simulink model "ADCS_onOrbit"  (R2024b)
settings: Solver=ode4  StartTime=0.0  StopTime=tspan  FixedStep=1  RelTol=1e-5
values from neighbouring files (symbols this model uses):
  A_list = [10*30; 10*30; 10*10; 10*30; 10*30; 10*10] * 1e-04    [acsLoadParameters.m]
  A_m = eye(3)    [acsLoadParameters.m]
  A_w = eye(3)    [acsLoadParameters.m]
  CD = 2.3    [acsLoadParameters.m]
  COP = [xAxis/2   0          0 ... (first row only)    [acsLoadParameters.m]
  dYear = decyear(YYYY,MM,DD)    [acsLoadParameters.m]
  e = 6.91944e-15    [acsLoadParameters.m]
  eta = 0.3    [acsLoadParameters.m]
  inc = 97.4377    [acsLoadParameters.m]
  J_body = [I_x 0 0; 0 I_y 0; 0 0 I_z]    [acsLoadParameters.m]
  J_wheels = [12894 0 0; 0 12774 0; 0 0 18389] * 1e-09    [acsLoadParameters.m]
  JD0 = juliandate(YYYY,MM,DD,HH,MIN,SEC)    [acsLoadParameters.m]
  K_d = 0.008    [acsLoadParameters.m]
  K_p = 0.003    [acsLoadParameters.m]
  K_w = 50e4    (= 500000)    [acsLoadParameters.m]
  m = 4    [acsLoadParameters.m]
  mag_moment = [0.005; 0.005; 0.005]    [acsLoadParameters.m]
  mu = 398600.4418    [acsLoadParameters.m]
  n_list = [1 0 0; 0 1 0; 0 0 1; -1 0 0; 0 -1 0; 0 0 -1]    [acsLoadParameters.m]
  omega = 0    [acsLoadParameters.m]    (also in orbit_plot_sfcn.m = block.InputPort(4).Data(:))
  p = 0.00000451    (= 4.51e-06)    [acsLoadParameters.m]    (also in cubesat_attitude_sfcn.m = ud.cubePos)
  P_0 = 0.0000001 * eye(7)    [acsLoadParameters.m]
  period = sqrt((4* pi^2 * semimajor_axis^3)/(mu))    [acsLoadParameters.m]
  q_ini = [0; 0; 0; 1]    [acsLoadParameters.m]
  raan = 226.816    [acsLoadParameters.m]
  rE = 6378.14    [acsLoadParameters.m]
  semimajor_axis = rE + h_apogee    (= 6913.14)    [acsLoadParameters.m]
  sigma_B_b = 0.05 * [1; 1; 1]    [acsLoadParameters.m]
  sigma_drift = 0.05 * [1; 1; 1] * 0    [acsLoadParameters.m]
  sigma_n = (0.05) * [1; 1; 1] * 0    [acsLoadParameters.m]
  sigma_S_b = 0.05 * [1; 1; 1]    [acsLoadParameters.m]
  tau = 300    [ATT_EKF_DOT.m]    (also in acsLoadParameters.m)
  true_anomaly = 0.0994843    [acsLoadParameters.m]
  w_b_ini = [0; 0.1; 0.1]    [acsLoadParameters.m]
  w_bias_0 = 0.0001 * [1; 1; 1] * 0    [acsLoadParameters.m]
  w_w_ini = [0; 0; 0]    [acsLoadParameters.m]
  wE = [0 0 15.04*(pi/180)*(1/3600)]    [acsLoadParameters.m]
undefined symbols (not defined in the file or in its folder): WMM2020
libraries: simulink_extras x13, matrix_library x9, sharedtransform x7, aerolibgravity2 x1, aerolibutil x1
(part 2 of 3)

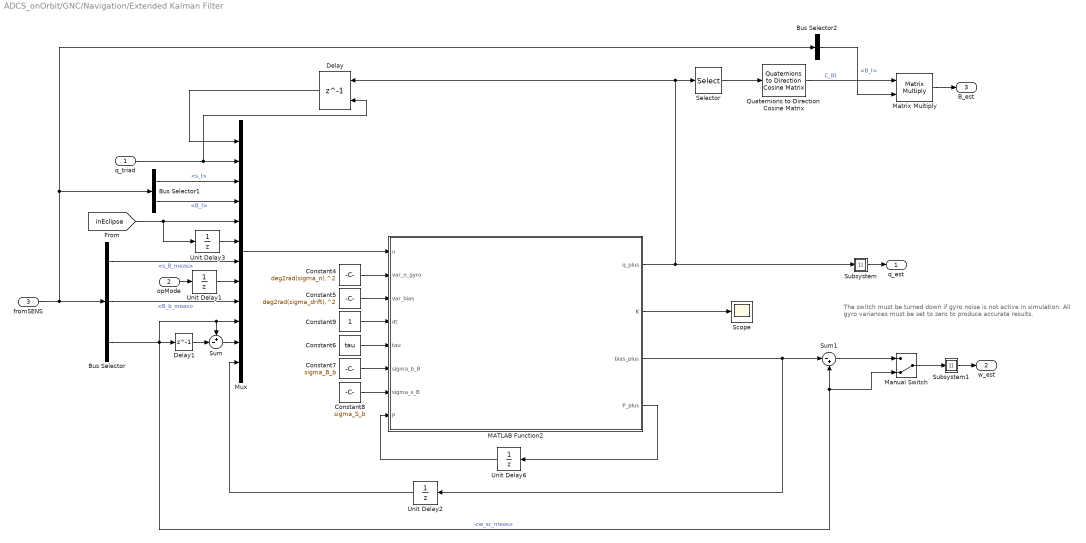
== system ADCS_onOrbit/GNC/Navigation/Extended Kalman Filter ==
  note: The switch must be turned down if gyro noise is not active in simulation.
      | All gyro variances must be set to zero to produce accurate results.
  q_triad : Inport
  opMode : Inport  Port=2
  fromSENS : Inport  Port=3
  Bus Selector : BusSelector  OutputSignals=s_B_meas,B_b_meas,w_sc_meas
  Bus Selector1 : BusSelector  OutputSignals=s_I,B_I
  Bus Selector2 : BusSelector  OutputSignals=B_I
  Constant4 : Constant  Value=deg2rad(sigma_n).^2
  Constant5 : Constant  Value=deg2rad(sigma_drift).^2
  Constant6 : Constant  Value=tau
  Constant7 : Constant  Value=sigma_B_b
  Constant8 : Constant  Value=sigma_S_b
  Constant9 : Constant
  Delay : Delay  DelayLength=1  InitialConditionSource=Input port  InitialCondition=q_ini
      settings: InputPortMap=u0,p4
  Delay1 : Delay  DelayLength=1  InitialCondition=w_b_ini
  MATLAB Function2 : MATLAB Function  TreatAsAtomicUnit=on
  Manual Switch : ManualSwitch  CurrentSetting=0
  Matrix Multiply : Product  Multiplication=Matrix(*)
  Mux : Mux  Inputs=12
  Quaternions to Direction Cosine Matrix : sharedtransform/Quaternions to  Direction Cosine Matrix  aMode=aMode
      settings: LibrarySourceBlock=|
      | aerolibtransform2/Quaternions to
      | Direction Cosine Matrix
  Scope : Scope
  Selector : Selector  InputPortWidth=4  IndexOptions=Index vector (dialog)  Indices=[4 1 2 3]  OutputSizes=1
  Subsystem : Subsystem
  Subsystem1 : Subsystem
  Sum : Sum  Inputs=+-|
  Sum1 : Sum  Inputs=|-+
  Unit Delay1 : UnitDelay  InitialCondition=-1  SampleTime=-1  HasFrameUpgradeWarning=on
  Unit Delay2 : UnitDelay  InitialCondition=w_bias_0  SampleTime=-1  HasFrameUpgradeWarning=on
  Unit Delay3 : UnitDelay  InitialCondition=-1  SampleTime=-1  HasFrameUpgradeWarning=on
  Unit Delay6 : UnitDelay  InitialCondition=P_0  SampleTime=-1  HasFrameUpgradeWarning=on
  q_est : Outport
  w_est : Outport  Port=2
  B_est : Outport  Port=3
  wires:
  [inEclipse] -> Unit Delay3/1, Mux/5
  fromSENS/1 -> Bus Selector1/1, Bus Selector2/1, Bus Selector/1
  MATLAB Function2/1(q_plus) -> Subsystem/1(q), Selector/1, Delay/1
  Sum1/1 -> Manual Switch/1
  Bus Selector/1 -> Mux/7  "<s_B_meas>"
  Bus Selector/2 -> Mux/9  "<B_b_meas>"
  Bus Selector1/1 -> Mux/3  "<s_I>"
  Bus Selector1/2 -> Mux/4  "<B_I>"
  Unit Delay3/1 -> Mux/6
  Delay/1 -> Mux/1
  q_triad/1 -> Delay/2, Mux/2
  opMode/1 -> Unit Delay1/1
  Unit Delay1/1 -> Mux/8
  Bus Selector/3 -> Delay1/1, Sum1/2, Manual Switch/2, Sum/1, Mux/10  "<w_sc_meas>"
  Sum/1 -> Mux/11
  Delay1/1 -> Sum/2
  MATLAB Function2/3(bias_plus) -> Unit Delay2/1, Sum1/1
  Unit Delay2/1 -> Mux/12
  Mux/1 -> MATLAB Function2/1(u)
  MATLAB Function2/4(P_plus) -> Unit Delay6/1
  Constant4/1 -> MATLAB Function2/2(var_n_gyro)
  Constant5/1 -> MATLAB Function2/3(var_bias)
  Constant6/1 -> MATLAB Function2/5(tau)
  Constant7/1 -> MATLAB Function2/6(sigma_b_B)
  Constant8/1 -> MATLAB Function2/7(sigma_s_B)
  Constant9/1 -> MATLAB Function2/4(dt)
  MATLAB Function2/2(K) -> Scope/1
  Selector/1 -> Quaternions to Direction Cosine Matrix/1
  Quaternions to Direction Cosine Matrix/1 -> Matrix Multiply/1  "C_BI"
  Bus Selector2/1 -> Matrix Multiply/2  "<B_I>"
  Matrix Multiply/1 -> B_est/1
  Subsystem/1(Out1) -> q_est/1
  Subsystem1/1(Out1) -> w_est/1
  Unit Delay6/1 -> MATLAB Function2/8(P)
  Manual Switch/1 -> Subsystem1/1(In1)

== system ADCS_onOrbit/GNC/Navigation/TRIAD Determination ==
  fromSENS : Inport
  Bus Selector : BusSelector  OutputSignals=s_I,B_I,s_B_meas,B_b_meas
  Direction Cosine Matrix to Quaternions : sharedtransform/Direction Cosine Matrix  to Quaternions  aMode=0  action=None  tolerance=eps(2)
      settings: LibrarySourceBlock=|
      | aerolibtransform2/Direction Cosine Matrix
      | to Quaternions
  MATLAB Function1 : MATLAB Function  TreatAsAtomicUnit=on
  Quaternion Continuity : Subsystem
      mask Display: disp('Quaternion\nContinuity');
  Selector2 : Selector  InputPortWidth=4  IndexOptions=Index vector (dialog)  Indices=[2 3 4 1]  OutputSizes=1
  q_det : Outport
  wires:
  Bus Selector/3 -> MATLAB Function1/3(s_b)  "<s_B_meas>"
  Bus Selector/4 -> MATLAB Function1/4(m_b)  "<B_b_meas>"
  fromSENS/1 -> Bus Selector/1
  MATLAB Function1/1(C_BI) -> Direction Cosine Matrix to Quaternions/1
  Direction Cosine Matrix to Quaternions/1 -> Selector2/1
  Selector2/1 -> Quaternion Continuity/1(q)
  Quaternion Continuity/1(q_smooth) -> q_det/1
  Bus Selector/1 -> MATLAB Function1/1(s_I)  "<s_I>"
  Bus Selector/2 -> MATLAB Function1/2(m_I)  "<B_I>"

== system ADCS_onOrbit/GNC/Navigation/rad2deg ==
  In1 : Inport
  Gain : Gain  Gain=57.2958
  Out1 : Outport
  wires:
  In1/1 -> Gain/1
  Gain/1 -> Out1/1

== system ADCS_onOrbit/RWP/Environment/Variant Subsystem ==
  note: 1) Add Subsystem or Model blocks as valid variant choices.
      | 2) You cannot connect blocks at this level. At simulation, connectivity is automatically
      | determined, based on the active variant and port name matching.
  C_BI : Inport
  s : Inport  Port=2
  state : Inport  Port=3
  ENV : Subsystem  VariantControl=external_torques == true
  noENV : Subsystem  VariantControl=external_torques == false
  B_b : Outport
  T_ext : Outport  Port=2
  a_drag : Outport  Port=3
  B_I : Outport  Port=4

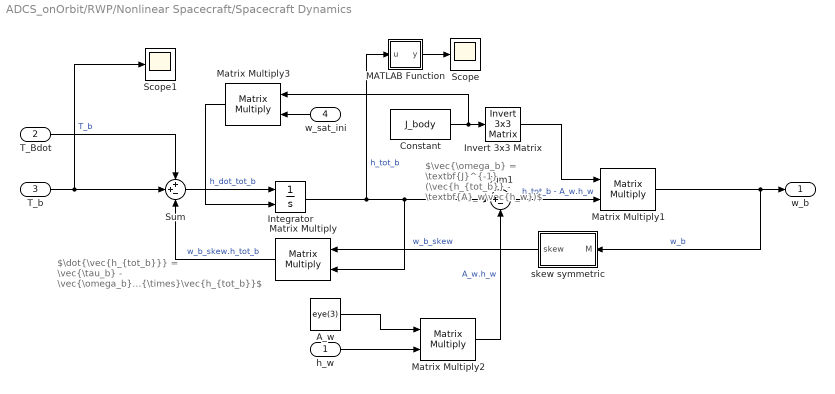
== system ADCS_onOrbit/RWP/Nonlinear Spacecraft/Spacecraft Dynamics ==
  note: $\dot{\vec{h_{tot_b}}} = \vec{\tau_b} - \vec{\omega_b}^{\times}\vec{h_{tot_b}}$
  note: $\vec{\omega_b} = \textbf{J}^{-1} (\vec{h_{tot_b}} - \textbf{A}_w\vec{h_w})$
  h_w : Inport
  T_Bdot : Inport  Port=2
  T_b : Inport  Port=3
  w_sat_ini : Inport  Port=4
  A_w : Constant  Value=eye(3)  VectorParams1D=off
  Constant : Constant  Value=J_body
  Integrator : Integrator  InitialConditionSource=external
  Invert 3x3 Matrix : aerolibutil/Invert  3x3 Matrix
  MATLAB Function : MATLAB Function  TreatAsAtomicUnit=on
  Matrix Multiply{,1..3} (4 alike) : Product  Multiplication=Matrix(*)
  Scope : Scope
  Scope1 : Scope
  Sum : Sum  Inputs=++-
  Sum1 : Sum  Inputs=|+-
  skew symmetric : MATLAB Function  TreatAsAtomicUnit=on
  w_b : Outport
  wires:
  Matrix Multiply2/1 -> Sum1/2  "A_w.h_w"
  A_w/1 -> Matrix Multiply2/1
  skew symmetric/1(skew) -> Matrix Multiply/1  "w_b_skew"
  Matrix Multiply1/1 -> w_b/1, skew symmetric/1(M)  "w_b"
  Invert 3x3 Matrix/1 -> Matrix Multiply1/1
  Constant/1 -> Matrix Multiply3/1, Invert 3x3 Matrix/1
  Sum1/1 -> Matrix Multiply1/2  "h_tot_b - A_w.h_w"
  h_w/1 -> Matrix Multiply2/2
  T_b/1 -> Scope1/1, Sum/2  "T_b"
  Matrix Multiply/1 -> Sum/3  "w_b_skew.h_tot_b"
  Sum/1 -> Integrator/1  "h_dot_tot_b"
  Integrator/1 -> MATLAB Function/1(u), Sum1/1, Matrix Multiply/2  "h_tot_b"
  w_sat_ini/1 -> Matrix Multiply3/2
  Matrix Multiply3/1 -> Integrator/2
  T_Bdot/1 -> Sum/1
  MATLAB Function/1(y) -> Scope/1

== system ADCS_onOrbit/RWP/Nonlinear Spacecraft/Spacecraft Kinematics ==
  note: Quaternion Kinematics Equation:
      | $\dot{\textbf{q}} = \frac{1}{2} \Omega (\vec\omega) \textbf{q}$
  w : Inport
  q_ini : Inport  Port=2
  Gain : Gain  Gain=1/2
  Integrator1 : Integrator  InitialConditionSource=external  InitialCondition=[1 0 0 0]
  MATLAB Function : MATLAB Function  TreatAsAtomicUnit=on
  Matrix Multiply3 : Product  Multiplication=Matrix(*)
  Quaternion Normalize : MATLAB Function  TreatAsAtomicUnit=on
  q : Outport
  wires:
  Matrix Multiply3/1 -> Integrator1/1  "dq/dt"
  MATLAB Function/1(OMEGA) -> Matrix Multiply3/1
  Gain/1 -> Matrix Multiply3/2
  q_ini/1 -> Integrator1/2
  Integrator1/1 -> Quaternion Normalize/1(q)  "q"
  w/1 -> MATLAB Function/1(w)
  Quaternion Normalize/1(q_norm) -> q/1, Gain/1

== system ADCS_onOrbit/RWP/Nonlinear Spacecraft/Subsystem ==
  q : Inport
  MATLAB Function : MATLAB Function  TreatAsAtomicUnit=on
  Radians to Degrees : simulink_extras/Transformations/Radians to Degrees
  Radians to Degrees1 : simulink_extras/Transformations/Radians to Degrees
  Radians to Degrees2 : simulink_extras/Transformations/Radians to Degrees
  To Workspace : ToWorkspace  VariableName=roll  SampleTime=-1
  To Workspace1 : ToWorkspace  VariableName=pitch  SampleTime=-1
  To Workspace2 : ToWorkspace  VariableName=yaw  SampleTime=-1
  Out1 : Outport
  tag scope: scAtt=global
  wires:
  q/1 -> MATLAB Function/1(q), Out1/1, [scAtt]
  MATLAB Function/3(pitch) -> Radians to Degrees1/1
  Radians to Degrees2/1 -> To Workspace2/1
  MATLAB Function/4(yaw) -> Radians to Degrees2/1
  MATLAB Function/2(roll) -> Radians to Degrees/1
  Radians to Degrees/1 -> To Workspace/1
  Radians to Degrees1/1 -> To Workspace1/1

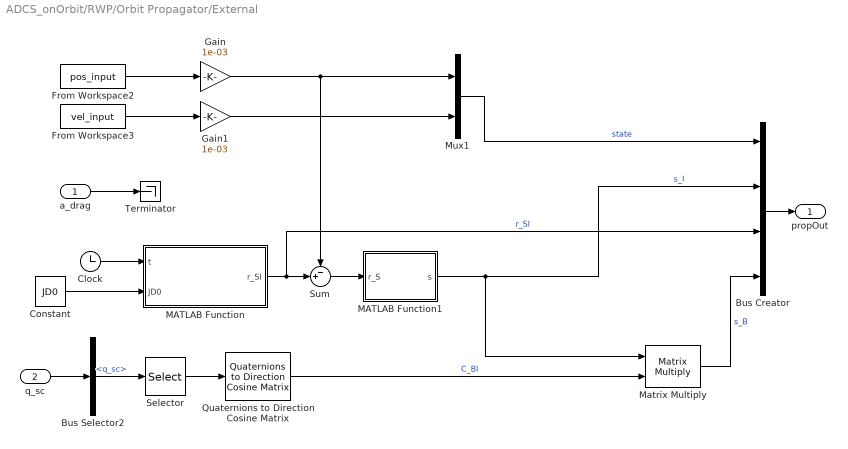
== system ADCS_onOrbit/RWP/Orbit Propagator/External ==
  a_drag : Inport
  q_sc : Inport  Port=2
  Bus Creator : BusCreator  Inputs=4
  Bus Selector2 : BusSelector  OutputSignals=q_sc
  Clock : Clock
  Constant : Constant  Value=JD0
  From Workspace2 : FromWorkspace  VariableName=pos_input
  From Workspace3 : FromWorkspace  VariableName=vel_input
  Gain : Gain  Gain=1e-03
  Gain1 : Gain  Gain=1e-03
  MATLAB Function : MATLAB Function  TreatAsAtomicUnit=on
  MATLAB Function1 : MATLAB Function  TreatAsAtomicUnit=on
  Matrix Multiply : Product  Multiplication=Matrix(*)
  Mux1 : Mux  Inputs=2
  Quaternions to Direction Cosine Matrix : sharedtransform/Quaternions to  Direction Cosine Matrix  aMode=aMode
      settings: LibrarySourceBlock=|
      | aerolibtransform2/Quaternions to
      | Direction Cosine Matrix
  Selector : Selector  InputPortWidth=4  IndexOptions=Index vector (dialog)  Indices=[4 1 2 3]  OutputSizes=1
  Sum : Sum  Inputs=-+|
  Terminator : Terminator
  propOut : Outport
  wires:
  Clock/1 -> MATLAB Function/1(t)
  From Workspace3/1 -> Gain1/1
  Gain/1 -> Sum/1, Mux1/1
  From Workspace2/1 -> Gain/1
  Sum/1 -> MATLAB Function1/1(r_S)
  Constant/1 -> MATLAB Function/2(JD0)
  Gain1/1 -> Mux1/2
  a_drag/1 -> Terminator/1
  MATLAB Function/1(r_SI) -> Bus Creator/3, Sum/2  "r_SI"
  MATLAB Function1/1(s) -> Matrix Multiply/1, Bus Creator/2  "s_I"
  Matrix Multiply/1 -> Bus Creator/4  "s_B"
  Bus Creator/1 -> propOut/1
  Mux1/1 -> Bus Creator/1  "state"
  Quaternions to Direction Cosine Matrix/1 -> Matrix Multiply/2  "C_BI"
  Selector/1 -> Quaternions to Direction Cosine Matrix/1
  q_sc/1 -> Bus Selector2/1
  Bus Selector2/1 -> Selector/1  "<q_sc>"

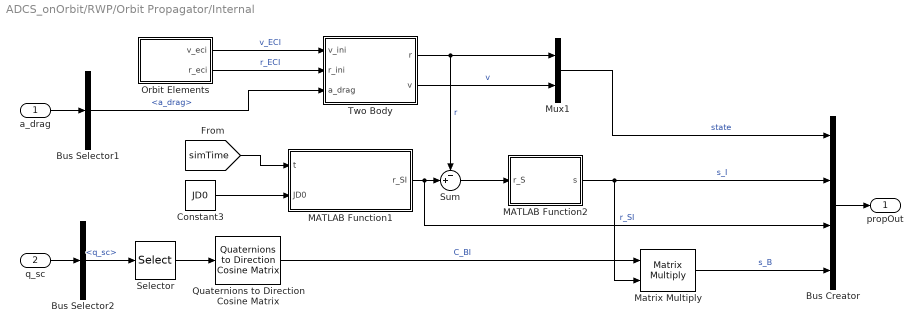
== system ADCS_onOrbit/RWP/Orbit Propagator/Internal ==
  a_drag : Inport
  q_sc : Inport  Port=2
  Bus Creator : BusCreator  Inputs=4
  Bus Selector1 : BusSelector  OutputSignals=a_drag
  Bus Selector2 : BusSelector  OutputSignals=q_sc
  Constant3 : Constant  Value=JD0
  MATLAB Function1 : MATLAB Function  TreatAsAtomicUnit=on
  MATLAB Function2 : MATLAB Function  TreatAsAtomicUnit=on
  Matrix Multiply : Product  Multiplication=Matrix(*)
  Mux1 : Mux  Inputs=2
  Orbit Elements : Subsystem
      mask Display: disp('OE2rv');
  Quaternions to Direction Cosine Matrix : sharedtransform/Quaternions to  Direction Cosine Matrix  aMode=aMode
      settings: LibrarySourceBlock=|
      | aerolibtransform2/Quaternions to
      | Direction Cosine Matrix
  Selector : Selector  InputPortWidth=4  IndexOptions=Index vector (dialog)  Indices=[4 1 2 3]  OutputSizes=1
  Sum : Sum  Inputs=-+|
  Two Body : Subsystem
      mask Display: disp('Two Body');
  propOut : Outport
  wires:
  Mux1/1 -> Bus Creator/1  "state"
  MATLAB Function1/1(r_SI) -> Bus Creator/3, Sum/2  "r_SI"
  Constant3/1 -> MATLAB Function1/2(JD0)
  [simTime] -> MATLAB Function1/1(t)
  Sum/1 -> MATLAB Function2/1(r_S)
  Orbit Elements/2(r_eci) -> Two Body/2(r_ini)  "r_ECI"
  Two Body/2(v) -> Mux1/2  "v"
  Two Body/1(r) -> Mux1/1, Sum/1  "r"
  a_drag/1 -> Bus Selector1/1
  Orbit Elements/1(v_eci) -> Two Body/1(v_ini)  "v_ECI"
  q_sc/1 -> Bus Selector2/1
  Selector/1 -> Quaternions to Direction Cosine Matrix/1
  Quaternions to Direction Cosine Matrix/1 -> Matrix Multiply/1  "C_BI"
  MATLAB Function2/1(s) -> Matrix Multiply/2, Bus Creator/2  "s_I"
  Matrix Multiply/1 -> Bus Creator/4  "s_B"
  Bus Selector2/1 -> Selector/1  "<q_sc>"
  Bus Selector1/1 -> Two Body/3(a_drag)  "<a_drag>"
  Bus Creator/1 -> propOut/1

== system ADCS_onOrbit/RWP/Subsystem/Subsystem1 ==
  In1 : Inport
  Out1 : Outport
  tag scope: w_w=global
  wires:
  In1/1 -> Out1/1, [w_w]

== system ADCS_onOrbit/RWP/Subsystem/Subsystem2 ==
  In1 : Inport
  Out1 : Outport
  tag scope: s_I=global
  wires:
  In1/1 -> [s_I], Out1/1

== system ADCS_onOrbit/GNC/Guidance/Nadir Pointing/Quaternion Continuity ==
  q : Inport
  MATLAB Function2 : MATLAB Function  TreatAsAtomicUnit=on
  Unit Delay1 : UnitDelay  InitialCondition=[0 0 0 1]'  SampleTime=-1  HasFrameUpgradeWarning=on
  q_smooth : Outport
  wires:
  MATLAB Function2/1(q_smooth) -> q_smooth/1, Unit Delay1/1
  Unit Delay1/1 -> MATLAB Function2/2(q_prev)
  q/1 -> MATLAB Function2/1(q)

== system ADCS_onOrbit/GNC/Guidance/Sun Pointing/Quaternion Continuity ==
  q : Inport
  MATLAB Function2 : MATLAB Function  TreatAsAtomicUnit=on
  Unit Delay1 : UnitDelay  InitialCondition=[0 0 0 1]'  SampleTime=-1  HasFrameUpgradeWarning=on
  q_smooth : Outport
  wires:
  MATLAB Function2/1(q_smooth) -> q_smooth/1, Unit Delay1/1
  Unit Delay1/1 -> MATLAB Function2/2(q_prev)
  q/1 -> MATLAB Function2/1(q)

== system ADCS_onOrbit/GNC/Guidance/Target Pointing/Quaternion Continuity ==
  q : Inport
  MATLAB Function2 : MATLAB Function  TreatAsAtomicUnit=on
  Unit Delay1 : UnitDelay  InitialCondition=[0 0 0 1]'  SampleTime=-1  HasFrameUpgradeWarning=on
  q_smooth : Outport
  wires:
  MATLAB Function2/1(q_smooth) -> q_smooth/1, Unit Delay1/1
  Unit Delay1/1 -> MATLAB Function2/2(q_prev)
  q/1 -> MATLAB Function2/1(q)

== system ADCS_onOrbit/GNC/Navigation/Extended Kalman Filter/Subsystem ==
  q : Inport
  MATLAB Function : MATLAB Function  TreatAsAtomicUnit=on
  Radians to Degrees : simulink_extras/Transformations/Radians to Degrees
  Radians to Degrees1 : simulink_extras/Transformations/Radians to Degrees
  Radians to Degrees2 : simulink_extras/Transformations/Radians to Degrees
  To Workspace : ToWorkspace  VariableName=rollEKF  SampleTime=-1
  To Workspace1 : ToWorkspace  VariableName=pitchEKF  SampleTime=-1
  To Workspace2 : ToWorkspace  VariableName=yawEKF  SampleTime=-1
  Out1 : Outport
  tag scope: rpy=global
  wires:
  q/1 -> MATLAB Function/1(q), Out1/1
  MATLAB Function/3(pitch) -> Radians to Degrees1/1
  Radians to Degrees2/1 -> To Workspace2/1
  MATLAB Function/4(yaw) -> Radians to Degrees2/1
  MATLAB Function/2(roll) -> Radians to Degrees/1
  Radians to Degrees/1 -> To Workspace/1
  Radians to Degrees1/1 -> To Workspace1/1
  MATLAB Function/1(rpy) -> [rpy]  "rpy"

== system ADCS_onOrbit/GNC/Navigation/Extended Kalman Filter/Subsystem1 ==
  In1 : Inport
  Out1 : Outport
  tag scope: w_body=global
  wires:
  In1/1 -> Out1/1, [w_body]

== system ADCS_onOrbit/GNC/Navigation/TRIAD Determination/Quaternion Continuity ==
  q : Inport
  MATLAB Function2 : MATLAB Function  TreatAsAtomicUnit=on
  Unit Delay1 : UnitDelay  InitialCondition=[0 0 0 1]'  SampleTime=-1  HasFrameUpgradeWarning=on
  q_smooth : Outport
  wires:
  MATLAB Function2/1(q_smooth) -> q_smooth/1, Unit Delay1/1
  Unit Delay1/1 -> MATLAB Function2/2(q_prev)
  q/1 -> MATLAB Function2/1(q)

== system ADCS_onOrbit/RWP/Environment/Variant Subsystem/ENV ==
  C_BI : Inport
  s : Inport  Port=2
  state : Inport  Port=3
  Drag : Subsystem
  Gravity Gradient : Subsystem
  Mag Torque : Subsystem
  Selector : Selector  InputPortWidth=6  IndexOptions=Index vector (dialog)  Indices=[1 2 3]  OutputSizes=1
  Selector1 : Selector  InputPortWidth=6  IndexOptions=Index vector (dialog)  Indices=[4 5 6]  OutputSizes=1
  Solar Radiation Pressure : Subsystem
  Sum : Sum  Inputs=++++
  B_b : Outport
  T_ext : Outport  Port=2
  a_drag : Outport  Port=3
  B_I : Outport  Port=4
  wires:
  Drag/2(a_drag) -> a_drag/1
  C_BI/1 -> Solar Radiation Pressure/1(C_BI), Drag/3(C_BI), Gravity Gradient/2(C_BI), Mag Torque/2(C_BI)
  Selector1/1 -> Drag/2(v_ECI)  "vel"
  Gravity Gradient/1(T_g) -> Sum/3
  Sum/1 -> T_ext/1  "External Torque"
  Mag Torque/1(T_mag) -> Sum/4
  Drag/1(T_atm) -> Sum/2
  Selector/1 -> Drag/1(r_ECI), Gravity Gradient/1(r_ECI), Mag Torque/1(r_ECI)  "pos"
  s/1 -> Solar Radiation Pressure/2(s)
  Mag Torque/2(B_b) -> B_b/1
  Solar Radiation Pressure/1(T_SRP) -> Sum/1
  state/1 -> Selector1/1, Selector/1
  Mag Torque/3(B_I) -> B_I/1

== system ADCS_onOrbit/RWP/Environment/Variant Subsystem/noENV ==
  C_BI : Inport
  s : Inport  Port=2
  state : Inport  Port=3
  Constant : Constant  Value=[0; 0; 0]  VectorParams1D=off
  Constant1 : Constant  Value=[0; 0; 0]
  Mag Torque : Subsystem
  Selector : Selector  InputPortWidth=6  IndexOptions=Index vector (dialog)  Indices=[1 2 3]  OutputSizes=1
  Terminator : Terminator
  Terminator1 : Terminator
  B_b : Outport
  T_ext : Outport  Port=2
  a_drag : Outport  Port=3
  B_I : Outport  Port=4
  wires:
  Constant1/1 -> a_drag/1
  Mag Torque/1(T_mag) -> Terminator1/1
  s/1 -> Terminator/1
  C_BI/1 -> Mag Torque/2(C_BI)
  Selector/1 -> Mag Torque/1(r_ECI)  "pos"
  state/1 -> Selector/1
  Constant/1 -> T_ext/1
  Mag Torque/2(B_b) -> B_b/1
  Mag Torque/3(B_I) -> B_I/1

== system ADCS_onOrbit/RWP/Orbit Propagator/Internal/Orbit Elements ==
  Constant : Constant  Value=semimajor_axis
  Constant1 : Constant  Value=e
  Constant2 : Constant  Value=inc
  Constant3 : Constant  Value=raan
  Constant4 : Constant  Value=omega
  Constant5 : Constant  Value=true_anomaly
  Constant6 : Constant  Value=mu
  Degrees to Radians{,1..3} (4 alike) : simulink_extras/Transformations/Degrees to Radians
  oe2rv : MATLAB Function  TreatAsAtomicUnit=on
  v_eci : Outport
  r_eci : Outport  Port=2
  wires:
  Degrees to Radians1/1 -> oe2rv/4(RAAN)
  Constant3/1 -> Degrees to Radians1/1
  Constant1/1 -> oe2rv/2(e)
  Degrees to Radians3/1 -> oe2rv/6(nu)
  Constant5/1 -> Degrees to Radians3/1
  Constant2/1 -> Degrees to Radians/1
  Constant4/1 -> Degrees to Radians2/1
  Degrees to Radians/1 -> oe2rv/3(i)
  Degrees to Radians2/1 -> oe2rv/5(omega)
  oe2rv/1(r_eci) -> r_eci/1
  oe2rv/2(v_eci) -> v_eci/1
  Constant/1 -> oe2rv/1(a)
  Constant6/1 -> oe2rv/7(mu)

== system ADCS_onOrbit/RWP/Orbit Propagator/Internal/Two Body ==
  v_ini : Inport
  r_ini : Inport  Port=2
  a_drag : Inport  Port=3
  Constant : Constant  Value=mu
  Constant1 : Constant  Value=rE
  Integrator2 : Integrator  InitialConditionSource=external
  Integrator3 : Integrator  InitialConditionSource=external
  MATLAB Function1 : MATLAB Function  TreatAsAtomicUnit=on
  MATLAB Function3 : MATLAB Function  TreatAsAtomicUnit=on
  Sum1 : Sum  Inputs=+++
  r : Outport
  v : Outport  Port=2
  wires:
  Constant/1 -> MATLAB Function3/2(mu), MATLAB Function1/2(mu)
  v_ini/1 -> Integrator2/2
  Integrator2/1 -> Integrator3/1, v/1  "r"
  r_ini/1 -> Integrator3/2
  MATLAB Function3/1(a_j2) -> Sum1/3  "a_J2"
  MATLAB Function1/1(a_I) -> Sum1/2
  Sum1/1 -> Integrator2/1
  Integrator3/1 -> r/1, MATLAB Function1/1(r_I), MATLAB Function3/1(r)  "r"
  a_drag/1 -> Sum1/1
  Constant1/1 -> MATLAB Function3/3(rE)

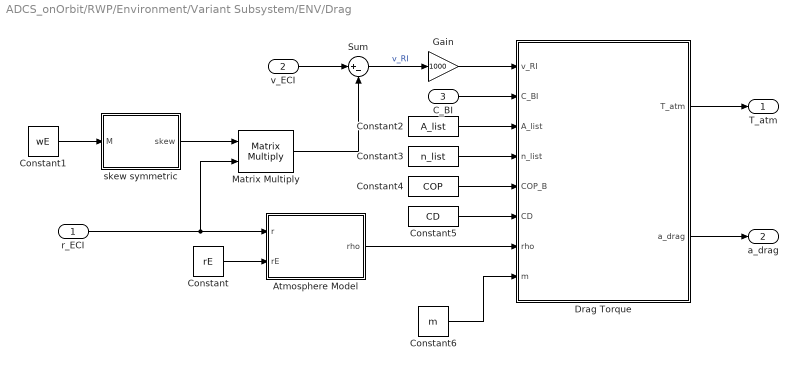
== system ADCS_onOrbit/RWP/Environment/Variant Subsystem/ENV/Drag ==
  r_ECI : Inport
  v_ECI : Inport  Port=2
  C_BI : Inport  Port=3
  Atmosphere Model : MATLAB Function  TreatAsAtomicUnit=on
  Constant : Constant  Value=rE
  Constant1 : Constant  Value=wE
  Constant2 : Constant  Value=A_list
  Constant3 : Constant  Value=n_list
  Constant4 : Constant  Value=COP
  Constant5 : Constant  Value=CD
  Constant6 : Constant  Value=m
  Drag Torque : MATLAB Function  TreatAsAtomicUnit=on
  Gain : Gain  Gain=1000
  Matrix Multiply : Product  Multiplication=Matrix(*)
  Sum : Sum  Inputs=|+-
  skew symmetric : MATLAB Function  TreatAsAtomicUnit=on
  T_atm : Outport
  a_drag : Outport  Port=2
  wires:
  Drag Torque/2(a_drag) -> a_drag/1
  Constant6/1 -> Drag Torque/8(m)
  Atmosphere Model/1(rho) -> Drag Torque/7(rho)
  Constant5/1 -> Drag Torque/6(CD)
  Constant4/1 -> Drag Torque/5(COP_B)
  Constant3/1 -> Drag Torque/4(n_list)
  Constant2/1 -> Drag Torque/3(A_list)
  C_BI/1 -> Drag Torque/2(C_BI)
  Gain/1 -> Drag Torque/1(v_RI)
  Sum/1 -> Gain/1  "v_RI"
  v_ECI/1 -> Sum/1
  Matrix Multiply/1 -> Sum/2
  Drag Torque/1(T_atm) -> T_atm/1
  skew symmetric/1(skew) -> Matrix Multiply/1
  Constant1/1 -> skew symmetric/1(M)
  Constant/1 -> Atmosphere Model/2(rE)
  r_ECI/1 -> Atmosphere Model/1(r), Matrix Multiply/2

== system ADCS_onOrbit/RWP/Environment/Variant Subsystem/ENV/Gravity Gradient ==
  r_ECI : Inport
  C_BI : Inport  Port=2
  Constant : Constant  Value=J_body
  Constant1 : Constant  Value=mu
  MATLAB Function : MATLAB Function  TreatAsAtomicUnit=on
  Matrix Multiply : Product  Multiplication=Matrix(*)
  Matrix Multiply1 : Product  Multiplication=Matrix(*)
  Matrix Multiply2 : Product  Multiplication=Matrix(*)
  Reshape1 : Reshape  OutputDimensionality=Customize  OutputDimensions=[3,1]
  skew symmetric : MATLAB Function  TreatAsAtomicUnit=on
  T_g : Outport
  wires:
  MATLAB Function/1(T_g) -> T_g/1
  Constant1/1 -> MATLAB Function/2(mu)
  Matrix Multiply2/1 -> MATLAB Function/3(r_skew_J_r)
  Matrix Multiply1/1 -> Matrix Multiply2/1
  Constant/1 -> Matrix Multiply1/2
  skew symmetric/1(skew) -> Matrix Multiply1/1
  C_BI/1 -> Matrix Multiply/1
  r_ECI/1 -> Matrix Multiply/2
  Matrix Multiply/1 -> Reshape1/1
  Reshape1/1 -> skew symmetric/1(M), MATLAB Function/1(r), Matrix Multiply2/2

== system ADCS_onOrbit/RWP/Environment/Variant Subsystem/ENV/Mag Torque ==
  r_ECI : Inport
  C_BI : Inport  Port=2
  Constant : Constant  Value=wE
  Constant1 : Constant  Value=dYear
  Constant4 : Constant  Value=mag_moment
  Demux1 : Demux  Outputs=2
  ECEF Position to LLA : ECEF2LLA
  Gain3 : Gain  Gain=1000
  MATLAB Function : MATLAB Function  TreatAsAtomicUnit=on
  MATLAB Function1 : MATLAB Function  TreatAsAtomicUnit=on
  Matrix Multiply : Product  Multiplication=Matrix(*)
  Subsystem2 : Subsystem
  T_mag : Outport
  B_b : Outport  Port=2
  B_I : Outport  Port=3
  wires:
  C_BI/1 -> MATLAB Function1/6(C_BI)
  Gain3/1 -> ECEF Position to LLA/1
  Matrix Multiply/1 -> Gain3/1
  r_ECI/1 -> Matrix Multiply/2
  MATLAB Function/1(C_IF) -> Matrix Multiply/1, Subsystem2/1(In1)
  Constant/1 -> MATLAB Function/1(wE)
  [simTime] -> MATLAB Function/2(t)
  ECEF Position to LLA/1 -> Demux1/1
  Demux1/1 -> MATLAB Function1/1(lat)
  Demux1/2 -> MATLAB Function1/2(lon)
  ECEF Position to LLA/2 -> MATLAB Function1/3(h)
  Constant1/1 -> MATLAB Function1/4(dYear)
  Constant4/1 -> MATLAB Function1/7(m)
  MATLAB Function1/1(b_I) -> B_I/1
  MATLAB Function1/2(b_B) -> B_b/1
  MATLAB Function1/3(T_m) -> T_mag/1
  Subsystem2/1(Out1) -> MATLAB Function1/5(C_IF)

== system ADCS_onOrbit/RWP/Environment/Variant Subsystem/ENV/Solar Radiation Pressure ==
  C_BI : Inport
  s : Inport  Port=2
  Constant1 : Constant  Value=p
  Constant2 : Constant  Value=eta
  Constant3 : Constant  Value=A_list
  Constant4 : Constant  Value=n_list
  Constant5 : Constant  Value=COP
  MATLAB Function2 : MATLAB Function  TreatAsAtomicUnit=on
  T_SRP : Outport
  wires:
  MATLAB Function2/1(T_SRP) -> T_SRP/1
  C_BI/1 -> MATLAB Function2/7(C_BI)
  Constant5/1 -> MATLAB Function2/6(COP)
  Constant4/1 -> MATLAB Function2/5(n_list)
  Constant3/1 -> MATLAB Function2/4(A_list)
  Constant2/1 -> MATLAB Function2/3(eta)
  Constant1/1 -> MATLAB Function2/2(p)
  s/1 -> MATLAB Function2/1(r_sun)

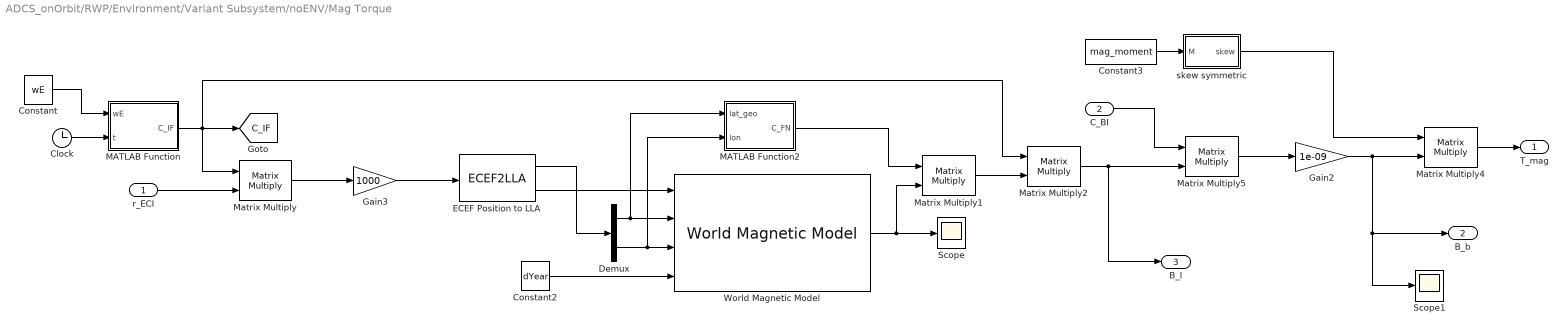
== system ADCS_onOrbit/RWP/Environment/Variant Subsystem/noENV/Mag Torque ==
  r_ECI : Inport
  C_BI : Inport  Port=2
  Clock : Clock
  Constant : Constant  Value=wE
  Constant2 : Constant  Value=dYear
  Constant3 : Constant  Value=mag_moment
  Demux : Demux  Outputs=2
  ECEF Position to LLA : ECEF2LLA
  Gain2 : Gain  Gain=1e-09
  Gain3 : Gain  Gain=1000
  MATLAB Function : MATLAB Function  TreatAsAtomicUnit=on
  MATLAB Function2 : MATLAB Function  TreatAsAtomicUnit=on
  Matrix Multiply{,1..2,4..5} (5 alike) : Product  Multiplication=Matrix(*)
  Scope : Scope
  Scope1 : Scope
  World Magnetic Model : aerolibgravity2/World Magnetic Model  model=WMM2020 (2020-2025)  customFile='WMM2020.COF'  units=Metric (MKS)  time_in=on  month=January  day=1  year=2020  action=Error  h_out=off  dec_out=off  inc_out=off  ti_out=off
  skew symmetric : MATLAB Function  TreatAsAtomicUnit=on
  T_mag : Outport
  B_b : Outport  Port=2
  B_I : Outport  Port=3
  tag scope: C_IF=global
  wires:
  Matrix Multiply5/1 -> Gain2/1
  C_BI/1 -> Matrix Multiply5/1
  Gain3/1 -> ECEF Position to LLA/1
  Demux/2 -> World Magnetic Model/3, MATLAB Function2/2(lon)
  Demux/1 -> World Magnetic Model/2, MATLAB Function2/1(lat_geo)
  ECEF Position to LLA/2 -> World Magnetic Model/1
  ECEF Position to LLA/1 -> Demux/1
  Matrix Multiply4/1 -> T_mag/1
  skew symmetric/1(skew) -> Matrix Multiply4/1
  Gain2/1 -> Matrix Multiply4/2, Scope1/1, B_b/1
  Constant3/1 -> skew symmetric/1(M)
  Matrix Multiply2/1 -> B_I/1, Matrix Multiply5/2
  Matrix Multiply1/1 -> Matrix Multiply2/2
  MATLAB Function2/1(C_FN) -> Matrix Multiply1/1
  World Magnetic Model/1 -> Scope/1, Matrix Multiply1/2
  Constant2/1 -> World Magnetic Model/4
  Matrix Multiply/1 -> Gain3/1
  r_ECI/1 -> Matrix Multiply/2
  MATLAB Function/1(C_IF) -> [C_IF], Matrix Multiply/1, Matrix Multiply2/1
  Constant/1 -> MATLAB Function/1(wE)
  Clock/1 -> MATLAB Function/2(t)

== system ADCS_onOrbit/RWP/Environment/Variant Subsystem/ENV/Mag Torque/Subsystem2 ==
  In1 : Inport
  Out1 : Outport
  tag scope: C_IF=global
  wires:
  In1/1 -> [C_IF], Out1/1

== matlab function ADCS_onOrbit/GNC/Guidance/Nadir Pointing/Quaternion Continuity/MATLAB Function2 ==
  data: q input; q_smooth output; q_prev input
function q_smooth = continuity(q, q_prev)

    if dot(q, q_prev) < 0
        q_smooth = -q;
    else
        q_smooth = q;
    end
end

== matlab function ADCS_onOrbit/GNC/Guidance/Sun Pointing/Quaternion Continuity/MATLAB Function2 ==
  data: q input; q_smooth output; q_prev input
function q_smooth = continuity(q, q_prev)

    if dot(q, q_prev) < 0
        q_smooth = -q;
    else
        q_smooth = q;
    end
end

== matlab function ADCS_onOrbit/RWP/Nonlinear Spacecraft/Spacecraft Kinematics/MATLAB Function ==
  data: w input; OMEGA output
function OMEGA = skew(w)

    w_1 = w(1,:);
    w_2 = w(2,:);
    w_3 = w(3,:);

    OMEGA = [0 w_3 -w_2 w_1
            -w_3 0 w_1 w_2
            w_2 -w_1 0 w_3
            -w_1 -w_2 -w_3 0];

end

== matlab function ADCS_onOrbit/GNC/Guidance/Target Pointing/MATLAB Function2 ==
  data: los input; C_BI output; r input; v input
function C_BI = fcn(los, r, v)

    los = los / norm(los);
    
    z_orb = los;

    y_orb = cross(v, r) / norm(cross(v,r)); % orbit normal
    y_orb = y_orb / norm(y_orb);

    x_orb = cross(y_orb, z_orb); 
    x_orb = x_orb / norm(x_orb);
    
    C_BI = [x_orb, y_orb, z_orb]';

end

== matlab function ADCS_onOrbit/GNC/Guidance/Target Pointing/Quaternion Continuity/MATLAB Function2 ==
  data: q input; q_smooth output; q_prev input
function q_smooth = continuity(q, q_prev)

    if dot(q, q_prev) < 0
        q_smooth = -q;
    else
        q_smooth = q;
    end
end

== matlab function ADCS_onOrbit/GNC/Error/Error Quaternion ==
  data: q input; delta_q output; q_d input
function delta_q = error_quaternion(q, q_d)

    delta_q = [q_d(4) q_d(3) -q_d(2) -q_d(1)
               -q_d(3) q_d(4) q_d(1) -q_d(2)
               q_d(2) -q_d(1) q_d(4) -q_d(3)
               q_d(1) q_d(2) q_d(3) q_d(4)] * q;

end

== matlab function ADCS_onOrbit/GNC/Error/MATLAB Function ==
  data: q_error input; theta_e output
function theta_e = pointing_error(q_error)

    q_error = q_error/norm(q_error);
    q4 = q_error(4,:);
    
    theta_e = rad2deg(2*acos(q4));

end

== matlab function ADCS_onOrbit/GNC/Guidance/Target Pointing/MATLAB Function3 ==
  data: q input; w_b output; q_dot input
function w_b = fcn(q, q_dot)

    E = q(1:3);     % vector part of quaternion
    n = q(4);       % scalar part

    E_skew = [  0     -E(3)   E(2);
              E(3)     0    -E(1);
             -E(2)   E(1)    0  ];

    % Construct 4x3 Omega matrix
    Omega = [0.5 * (n * eye(3) + E_skew);   
             -0.5 * E'];                   

    w_b = Omega \ q_dot;   % Use backslash for stability instead of inv()

end

== matlab function ADCS_onOrbit/GNC/Error/Subsystem/MATLAB Function1 ==
  data: q input; roll output; pitch output; yaw output
function [roll, pitch, yaw] = fcn(q)

    x = q(1);
    y = q(2);
    z = q(3);
    w = q(4);

    % Roll
    sinr_cosp = 2 * (w*x + y*z);
    cosr_cosp = 1 - 2 * (x^2 + y^2);
    roll = atan2(sinr_cosp, cosr_cosp);

    % Pitch
    sinp = 2 * (w * y - z * x);
    sinp = max(min(sinp, 1), -1);
    pitch = asin(sinp);

    % Yaw
    siny_cosp = 2 * (w * z + x * y);
    cosy_cosp = 1 - 2 * (y^2 + z^2);
    yaw = atan2(siny_cosp, cosy_cosp);


end

== matlab function ADCS_onOrbit/RWP/Nonlinear Spacecraft/Spacecraft Dynamics/MATLAB Function ==
  data: u input; y output
function y = fcn(u)

y = norm(u);

== matlab function ADCS_onOrbit/RWP/Environment/Variant Subsystem/ENV/Mag Torque/MATLAB Function1 ==
  data: lat input; b_I output; lon input; h input; dYear input; C_IF input; C_BI input; m input; b_B output; T_m output
function [b_I, b_B, T_m] = fcn(lat, lon, h, dYear, C_IF, C_BI, m)

    coder.extrinsic('wrldmagm');
    dYear = 2025.0;             % WMM2020 doesn't work for anything over 2025.0

    b = zeros(3,1);
    lat_geo = lat;

    m_skew = [0     m(3) -m(2)
             -m(3)  0     m(1)
              m(2) -m(1)  0  ];
    
    % World Magnetic Model
    [b, H, DEC, DIP, F] = wrldmagm(h, lat, lon, dYear,'2020');
    
    % Conversion to go from NED to ECEF
    sLat = sind(lat_geo);
    cLat = sind(lat_geo);

    sLon = sind(lon);
    cLon = cosd(lon);
 
    C_FN = [-sLat*cLon -sLat*sLon cLat; -sLon cLon 0; -cLat*cLon -cLat*sLon -sLat]';
    b_ECEF = C_FN * b;

    % Going from ECEF to ECI
    b_I = C_IF * b_ECEF;

    % Conversion to Body Frame
    b_B = C_BI * b_I;

    % Magnetic Torque
    T_m = m_skew * b_B * 1e-09;

end

== matlab function ADCS_onOrbit/RWP/Nonlinear Spacecraft/Spacecraft Kinematics/Quaternion Normalize ==
  data: q input; q_norm output
function q_norm = q_normalize(q)

q_norm = q/norm(q);

== matlab function ADCS_onOrbit/RWP/Environment/MATLAB Function ==
  data: u input; y output
function y = magnitude(u)

y = norm(u);

== matlab function ADCS_onOrbit/RWP/Environment/Variant Subsystem/ENV/Drag/Atmosphere Model ==
  data: rho output; r input; rE input
function rho = atmosphere(r, rE)

    z = norm(r)-rE;        % Altitude (km) 

    if 450 <= z && z < 500
        rho0 = 1.585e-12;   % kg/m³
        h0 = 450;   % km
        H = 60.828;  % km
    else
        rho0 = 6.967e-13;   % kg/m³
        h0 = 500;   % km
        H = 63.822;  % km
    end

    rho = rho0 * exp(-(z-h0)/H);    % in kg/m³

end

== matlab function ADCS_onOrbit/RWP/Environment/Variant Subsystem/ENV/Drag/Drag Torque ==
  data: v_RI input; C_BI input; A_list input; n_list input; COP_B input; CD input; T_atm output; rho input; a_drag output; m input
function [T_atm, a_drag] = drag_torque(v_RI, C_BI, A_list, n_list, COP_B, CD, rho, m)

    v_RI_hat = v_RI / norm(v_RI);     
    v_RI_mag = norm(v_RI);            
    T_atm = [0; 0; 0];
    F_drag = [0; 0; 0];
    a_drag = [0; 0; 0];

    for k = 1:length(A_list)
        n_k = n_list(k, :).';         
        A_k = A_list(k);              

        cos_alpha_k = dot(n_k, C_BI * v_RI_hat);

        if cos_alpha_k > 0
            F_k = - 0.5 * rho * CD * A_k * v_RI_mag^2 * cos_alpha_k * v_RI_hat;
        else 
            F_k = [0; 0; 0];
        end
        F_drag = F_drag + F_k;
        a_drag = F_drag/m;

        F_k_B = C_BI * F_k;
        COP_B_k = COP_B(k, :).';
        T_k = cross(COP_B_k, F_k_B);
        T_atm = T_atm + T_k;
    end

end

== matlab function ADCS_onOrbit/RWP/Environment/Variant Subsystem/ENV/Drag/skew symmetric ==
  data: M input; skew output
function skew = skew_matrix(M)

    skew = [0 M(3) -M(2)
            -M(3) 0 M(1)
            M(2) -M(1) 0];

end

== matlab function ADCS_onOrbit/RWP/Environment/Variant Subsystem/ENV/Gravity Gradient/MATLAB Function ==
  data: r input; mu input; T_g output; r_skew_J_r input
function T_g = T_g(r, mu, r_skew_J_r)

    T_g = (3*mu/norm(r)^5) * r_skew_J_r;

end

== matlab function ADCS_onOrbit/OBC/RES/MATLAB Function ==
  data: u input; y output
function y = magnitude(u)

y = norm(u);

== matlab function ADCS_onOrbit/GNC/Guidance/MATLAB Function ==
  data: R_s input; eclipse_entry output; r_sat input; r_E input; was_in_eclipse input; eclipse_exit output; is_in_eclipse output
function [eclipse_entry, eclipse_exit, is_in_eclipse] = fcn(R_s, r_sat, r_E, was_in_eclipse)

    % Convert input to numeric (if it came in as logical)
    if was_in_eclipse
        was = 1;
    else
        was = 0;
    end

    % Normalize sun vector
    s_hat = R_s / norm(R_s);

    % Projection of satellite position onto sun vector
    proj = dot(r_sat, s_hat);
    closest_point = proj * s_hat;

    % Perpendicular distance from Earth center to Sun-sat line
    d = norm(r_sat - closest_point);

    % Check if satellite is in eclipse
    if (d < r_E) && (proj < 0)
        is_in_eclipse = 1;
    else
        is_in_eclipse = 0;
    end

    % Detect eclipse entry
    if (was == 0) && (is_in_eclipse == 1)
        eclipse_entry = 1;
    else
        eclipse_entry = 0;
    end

    % Detect eclipse exit
    if (was == 1) && (is_in_eclipse == 0)
        eclipse_exit = 1;
    else
        eclipse_exit = 0;
    end

end

== matlab function ADCS_onOrbit/RWP/Environment/Variant Subsystem/ENV/Gravity Gradient/skew symmetric ==
  data: M input; skew output
function skew = skew_matrix(M)

    skew = [0 M(3) -M(2)
            -M(3) 0 M(1)
            M(2) -M(1) 0];

end

== matlab function ADCS_onOrbit/GNC/Guidance/Nadir Pointing/ECI to SB ==
  data: r input; C_BI output; v input
function C_BI = fcn(r, v)

    % Converts vectors in ECI to Spacecraft Body Frame

    r = r(:); v = v(:);
    
    z_orb = - r / norm(r);                  % nadir
    y_orb = cross(v, r) / norm(cross(v,r)); % orbit normal
    y_orb = y_orb / norm(y_orb);

    x_orb = cross(y_orb, z_orb); 
    x_orb = x_orb / norm(x_orb);

    C_BI = [x_orb, y_orb, z_orb]';
end

== matlab function ADCS_onOrbit/GNC/Guidance/Sequence Logic ==
  data: q_GC input; w_GC input; q_nadir input; q output; w_nadir input; q_sun input; w_sun input; t input; opMode input; in_eclipse input; w output; eclipse_exit input; mode output; t_eclipse_exit_prev input; t_eclipse_exit_out output
function [q, w, mode, t_eclipse_exit_out] = fcn(q_GC, w_GC, q_nadir, w_nadir, q_sun, w_sun, t, opMode, in_eclipse, eclipse_exit, t_eclipse_exit_prev)

    option = opMode;
    q = zeros(4,1);
    w = zeros(3,1);
    mode = 0;

    % Store new eclipse exit time if just exited
    if eclipse_exit == 1
        t_eclipse_exit_out = t;
    else
        t_eclipse_exit_out = t_eclipse_exit_prev;
    end

    % Manual override modes
    % For mission mode, detumble mode, desaturation mode and safemode
    if option ~= 1 && option ~= 2 && option ~= 3
        q = q_nadir;
        w = w_nadir;
        mode = 0;

    % For comms mode
    elseif option == 3
        q = q_GC;
        w = w_GC;
       
    % Idle mode
    elseif option == 1
        q = q_sun;
        w = w_sun;
        mode = 1;

    % Auto switch mode
    elseif option == 2
        if in_eclipse == 1
            q = q_sun;
            w = w_sun;
            mode = 1;
        else
            if t <= (t_eclipse_exit_out + 30*60)
                q = q_sun;
                w = w_sun;
                mode = 1;
            else
                q = q_nadir;
                w = w_nadir;
                mode = 0;
            end
        end
    end

end

== matlab function ADCS_onOrbit/RWP/Environment/Variant Subsystem/ENV/Mag Torque/MATLAB Function ==
  data: wE input; C_IF output; t input
function C_IF = fcn(wE, t)

    theta = wE(3) * t;

    C_IF = [cos(theta) sin(theta) 0; -sin(theta) cos(theta) 0; 0 0 1]';

end

== matlab function ADCS_onOrbit/GNC/Guidance/Sun Pointing/MATLAB Function ==
  data: q output; DCM input
function q = dcm2quat(DCM)
    A = DCM;
    q = zeros(4,1); % [q1; q2; q3; q4] — vector-first

    tr = trace(A);

    if tr > 0
        S = sqrt(tr + 1.0) * 2; % S = 4*q4
        q(4) = 0.25 * S;
        q(1) = (A(3,2) - A(2,3)) / S;
        q(2) = (A(1,3) - A(3,1)) / S;
        q(3) = (A(2,1) - A(1,2)) / S;
    elseif (A(1,1) > A(2,2)) && (A(1,1) > A(3,3))
        S = sqrt(1.0 + A(1,1) - A(2,2) - A(3,3)) * 2; % S = 4*q1
        q(1) = 0.25 * S;
        q(2) = (A(1,2) + A(2,1)) / S;
        q(3) = (A(1,3) + A(3,1)) / S;
        q(4) = (A(3,2) - A(2,3)) / S;
    elseif (A(2,2) > A(3,3))
        S = sqrt(1.0 + A(2,2) - A(1,1) - A(3,3)) * 2; % S = 4*q2
        q(1) = (A(1,2) + A(2,1)) / S;
        q(2) = 0.25 * S;
        q(3) = (A(2,3) + A(3,2)) / S;
        q(4) = (A(1,3) - A(3,1)) / S;
    else
        S = sqrt(1.0 + A(3,3) - A(1,1) - A(2,2)) * 2; % S = 4*q3
        q(1) = (A(1,3) + A(3,1)) / S;
        q(2) = (A(2,3) + A(3,2)) / S;
        q(3) = 0.25 * S;
        q(4) = (A(2,1) - A(1,2)) / S;
    end

    q = q / norm(q); % normalize
end

== matlab function ADCS_onOrbit/RWP/Environment/Variant Subsystem/ENV/Solar Radiation Pressure/MATLAB Function2 ==
  data: r_sun input; T_SRP output; p input; eta input; A_list input; n_list input; COP input; C_BI input
function T_SRP = fcn(r_sun, p, eta, A_list, n_list, COP, C_BI)

    T_SRP = [0; 0; 0];
    r_sun = r_sun(:);  % ensure column vector

    for k = 1:length(A_list)
        n_k = n_list(k, :)';          % column vector (3x1)
        A_k = A_list(k);              % scalar area

        cos_alpha_k = dot(n_k, C_BI * r_sun);  % scalar

        if cos_alpha_k > 0
            F_srp_k = -p * A_k * eta * cos_alpha_k * r_sun;  % vector (3x1)
        else
            F_srp_k = [0; 0; 0];
        end

        F_srp_k_B = C_BI * F_srp_k;
        COP_k = COP(k, :)';
        T_SRP_k = cross(COP_k, F_srp_k_B);

        T_SRP = T_SRP + T_SRP_k;
    end

end

== matlab function ADCS_onOrbit/ACT/Wheels + Magnetorquers/MATLAB Function ==
  data: T_c input; T_cmd output; wheelsEnabled input
function T_cmd = fcn(T_c, wheelsEnabled)

if wheelsEnabled == 1
    T_cmd = T_c;
else
    T_cmd = [0; 0; 0];
end

end

== matlab function ADCS_onOrbit/RWP/Environment/Variant Subsystem/noENV/Mag Torque/MATLAB Function ==
  data: wE input; C_IF output; t input
function C_IF = fcn(wE, t)

    theta = wE(3) * t;

    C_IF = [cos(theta) sin(theta) 0; -sin(theta) cos(theta) 0; 0 0 1]';

end

== matlab function ADCS_onOrbit/RWP/Environment/Variant Subsystem/noENV/Mag Torque/MATLAB Function2 ==
  data: lat_geo input; C_FN output; lon input
function C_FN = fcn(lat_geo, lon)

   sLat = sind(lat_geo);
   cLat = sind(lat_geo);

   sLon = sind(lon);
   cLon = cosd(lon);

   C_FN = [-sLat*cLon -sLat*sLon cLat; -sLon cLon 0; -cLat*cLon -cLat*sLon -sLat]';


end

== matlab function ADCS_onOrbit/GNC/Guidance/Sun Pointing/MATLAB Function2 ==
  data: s_i input; C_BI output
function C_BI = fcn(s_i)

    % Ecliptic notth pole
    epsilon = deg2rad(23.44);  % Obliquity of the ecliptic
    n_ecl = [0; -sin(epsilon); cos(epsilon)];

    x_b = s_i / norm(s_i);
    z_b = n_ecl - dot(n_ecl, x_b) * x_b; % Gram-Schmidt orthogonalization
    z_b = z_b / norm(z_b); 
    if dot(z_b, n_ecl) < 0
        z_b = -z_b; 
    end
    y_b = cross(z_b, x_b);
    
    C1 = [x_b y_b z_b];   

    theta = deg2rad(45);

    Rz = [cos(theta), -sin(theta), 0;
          sin(theta),  cos(theta), 0;
          0,           0,          1];
    
    C_BI = C1 * Rz';

end

== matlab function ADCS_onOrbit/RWP/Environment/Variant Subsystem/noENV/Mag Torque/skew symmetric ==
  data: M input; skew output
function skew = skew_matrix(M)

    skew = [0 M(3) -M(2)
            -M(3) 0 M(1)
            M(2) -M(1) 0];

end

== matlab function ADCS_onOrbit/GNC/Navigation/TRIAD Determination/Quaternion Continuity/MATLAB Function2 ==
  data: q input; q_smooth output; q_prev input
function q_smooth = continuity(q, q_prev)

    if dot(q, q_prev) < 0
        q_smooth = -q;
    else
        q_smooth = q;
    end
end

== matlab function ADCS_onOrbit/GNC/Navigation/TRIAD Determination/MATLAB Function1 ==
  data: s_I input; C_BI output; m_I input; s_b input; m_b input
function C_BI = fcn(s_I, m_I, s_b, m_b)

% Normalizing vectors
sI = s_I/norm(s_I);
sB = s_b/norm(s_b);
mI = m_I/norm(m_I);
mB = m_b/norm(m_b);

% Determining M_I 
r1 = sI;
r2 = cross(sI,mI)/norm(cross(sI,mI));
r3 = cross(r1, r2);
MI = [r1, r2, r3];

% Determining M_B
s1 = sB;
s2 = cross(sB,mB)/norm(cross(sB,mB));
s3 = cross(s1, s2);

MB = [s1, s2, s3]; 

C_BI = MB * transpose(MI);

end
